simulink model "pid_Subsystem"  (R2020b)
settings: Solver=VariableStepAuto  StartTime=0.0  StopTime=10.0  RelTol=1e-3
model workspace (MAT data in the model file):
  J = 0.01
  K = 0.01
  L = 0.5
  R = 1
  b = 0.1
settings Model: Creator=Lakshmi  LastModifiedBy=Lakshmi
settings DataIOCC: SaveOutput=off  SaveTime=off

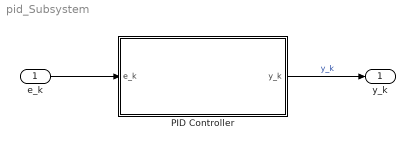
== system pid_Subsystem ==
  e_k : Inport  OutDataTypeStr=double  PortDimensions=1  SampleTime=0
  PID Controller : Subsystem  mask{Kp=370.0, Ki=50.0, Ts=0.001, Kd=-8.2490}
  y_k : Outport  OutDataTypeStr=double  PortDimensions=1  SampleTime=0
  wires:
  e_k/1 -> PID Controller/1(e_k)
  PID Controller/1(y_k) -> y_k/1  "y_k"

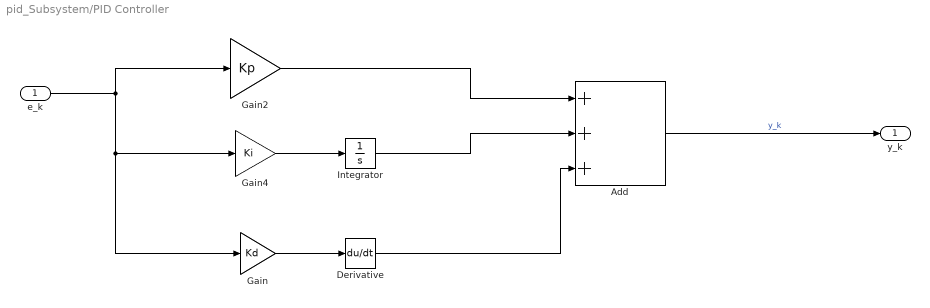
== system pid_Subsystem/PID Controller ==
  e_k : Inport
  Add : Sum  Inputs=+++
  Derivative : Derivative
  Gain : Gain  Gain=Kd
  Gain2 : Gain  Gain=Kp
  Gain4 : Gain  Gain=Ki
  Integrator : Integrator
  y_k : Outport
  wires:
  e_k/1 -> Gain/1, Gain4/1, Gain2/1
  Add/1 -> y_k/1  "y_k"
  Gain2/1 -> Add/1
  Gain/1 -> Derivative/1
  Gain4/1 -> Integrator/1
  Integrator/1 -> Add/2
  Derivative/1 -> Add/3
